simulink model "adi_jesd"  (R2021a)
settings: Solver=VariableStepAuto  StartTime=0.0  StopTime=10.0  RelTol=1e-3
libraries: xbsIndex_r4 x7
settings Model: Creator=jackh  LastModifiedBy=jackh

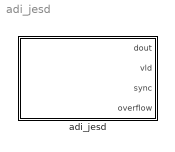
== system adi_jesd ==
  adi_jesd : Subsystem  Tag=xps:adi_jesd  mask(xsg_adi_jesd){fmc_port=0, adi_ip_path=/home/jackh/src/dsa2000-fpga/firmware/lib/adi_hdl/library, sample_rate_mhz=4800, block_diagram='adi_jesd_zynqusplus_adc_only.tcl', refclk_name=}
      mask prompts: fmc_port "FMC Port Number"; adi_ip_path "Path to ADI IP repository"; sample_rate_mhz "Sample rate (Msps)"; block_diagram "ADI JESD block diagram name"; refclk_name "REFCLK override. If set, should be a string such that <refclk_name>_n has a LOC defined in the platform's YAML file"
      mask init:
      | adi_jesd_init()
      mask Help: eval('xlWeb([getenv(''MLIB_ROOT''), ''\doc\html\sys_xsg_core_config\sys_xsg_core_config.html''])')

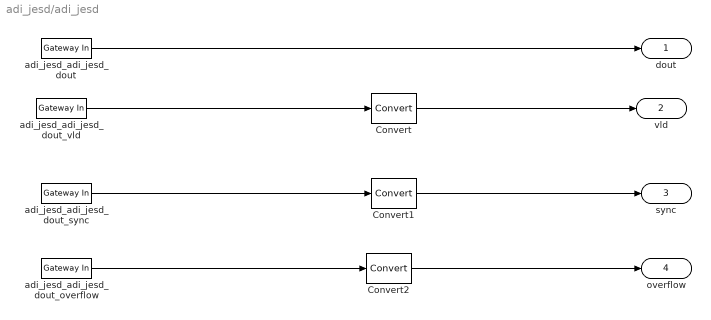
== system adi_jesd/adi_jesd ==
  Convert : xbsIndex_r4/Convert  gui_display_data_type=Boolean  arith_type=Boolean  n_bits=16  bin_pt=14  float_type=Single  exp_bits=8  fraction_bits=24  quantization=Truncate  overflow=Wrap  en=off  latency=0  pipeline=off  dbl_ovrd=off  block_type=convert
  Convert1 : xbsIndex_r4/Convert  gui_display_data_type=Boolean  arith_type=Boolean  n_bits=16  bin_pt=14  float_type=Single  exp_bits=8  fraction_bits=24  quantization=Truncate  overflow=Wrap  en=off  latency=0  pipeline=off  dbl_ovrd=off  block_type=convert
  Convert2 : xbsIndex_r4/Convert  gui_display_data_type=Boolean  arith_type=Boolean  n_bits=16  bin_pt=14  float_type=Single  exp_bits=8  fraction_bits=24  quantization=Truncate  overflow=Wrap  en=off  latency=0  pipeline=off  dbl_ovrd=off  block_type=convert
  adi_jesd_adi_jesd_dout : xbsIndex_r4/Gateway In  gui_display_data_type=Fixed-point  arith_type=Unsigned  n_bits=512  bin_pt=0  preci_type=Single  exp_width=8  frac_width=24  rows=1  columns=1  quantization=Truncate  overflow=Wrap  period=1  UseAsADC=off  ADCChannel='1'  interface=None  automatic_assignment=on  address_offset=hex2dec('00')  intf_name=''  intf_description=''  default_value=0  timing_constraint=None  locs_specified=off  LOCs={}  io_standard={}  inherit_from_input=off  hdl_port=on  dbl_ovrd=off  block_type=gatewayin
  adi_jesd_adi_jesd_dout_overflow : xbsIndex_r4/Gateway In  gui_display_data_type=Fixed-point  arith_type=Unsigned  n_bits=1  bin_pt=0  preci_type=Single  exp_width=8  frac_width=24  rows=1  columns=1  quantization=Truncate  overflow=Wrap  period=1  UseAsADC=off  ADCChannel='1'  interface=None  automatic_assignment=on  address_offset=hex2dec('00')  intf_name=''  intf_description=''  default_value=0  timing_constraint=None  locs_specified=off  LOCs={}  io_standard={}  inherit_from_input=off  hdl_port=on  dbl_ovrd=off  block_type=gatewayin
  adi_jesd_adi_jesd_dout_sync : xbsIndex_r4/Gateway In  gui_display_data_type=Fixed-point  arith_type=Unsigned  n_bits=1  bin_pt=0  preci_type=Single  exp_width=8  frac_width=24  rows=1  columns=1  quantization=Truncate  overflow=Wrap  period=1  UseAsADC=off  ADCChannel='1'  interface=None  automatic_assignment=on  address_offset=hex2dec('00')  intf_name=''  intf_description=''  default_value=0  timing_constraint=None  locs_specified=off  LOCs={}  io_standard={}  inherit_from_input=off  hdl_port=on  dbl_ovrd=off  block_type=gatewayin
  adi_jesd_adi_jesd_dout_vld : xbsIndex_r4/Gateway In  gui_display_data_type=Fixed-point  arith_type=Unsigned  n_bits=1  bin_pt=0  preci_type=Single  exp_width=8  frac_width=24  rows=1  columns=1  quantization=Truncate  overflow=Wrap  period=1  UseAsADC=off  ADCChannel='1'  interface=None  automatic_assignment=on  address_offset=hex2dec('00')  intf_name=''  intf_description=''  default_value=0  timing_constraint=None  locs_specified=off  LOCs={}  io_standard={}  inherit_from_input=off  hdl_port=on  dbl_ovrd=off  block_type=gatewayin
  dout : Outport  VectorParamsAs1DForOutWhenUnconnected=off
  vld : Outport  Port=2  VectorParamsAs1DForOutWhenUnconnected=off
  sync : Outport  Port=3  VectorParamsAs1DForOutWhenUnconnected=off
  overflow : Outport  Port=4  VectorParamsAs1DForOutWhenUnconnected=off
  wires:
  adi_jesd_adi_jesd_dout/1 -> dout/1
  adi_jesd_adi_jesd_dout_vld/1 -> Convert/1
  adi_jesd_adi_jesd_dout_sync/1 -> Convert1/1
  adi_jesd_adi_jesd_dout_overflow/1 -> Convert2/1
  Convert/1 -> vld/1
  Convert1/1 -> sync/1
  Convert2/1 -> overflow/1
